simulink model "blocks"  (R2017b)
settings: Solver=VariableStepAuto  StartTime=0.0  StopTime=10.0  RelTol=1e-3
undefined symbols (not defined in the file or in its folder): environment
libraries: sharedtransform x1, aerolibnav x1
settings Model: Creator=Martin  LastModifiedBy=Martin

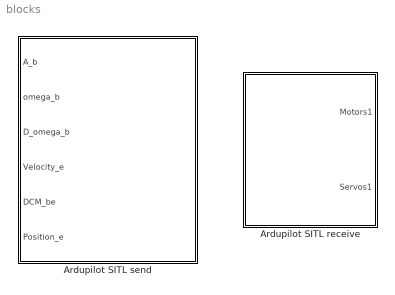
== system blocks ==
  Ardupilot SITL receive : Subsystem
  Ardupilot SITL send : Subsystem

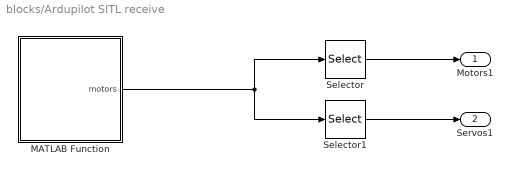
== system blocks/Ardupilot SITL receive ==
  MATLAB Function : MATLAB Function  TreatAsAtomicUnit=on  SystemSampleTime=0.02
  Selector : Selector  InputPortWidth=16  IndexOptions=Index vector (dialog)  Indices=sitl.output.motors  OutputSizes=1
  Selector1 : Selector  InputPortWidth=16  IndexOptions=Index vector (dialog)  Indices=sitl.output.servos  OutputSizes=1
  Motors1 : Outport
  Servos1 : Outport  Port=2
  wires:
  Selector1/1 -> Servos1/1
  Selector/1 -> Motors1/1
  MATLAB Function/1(motors) -> Selector1/1, Selector/1

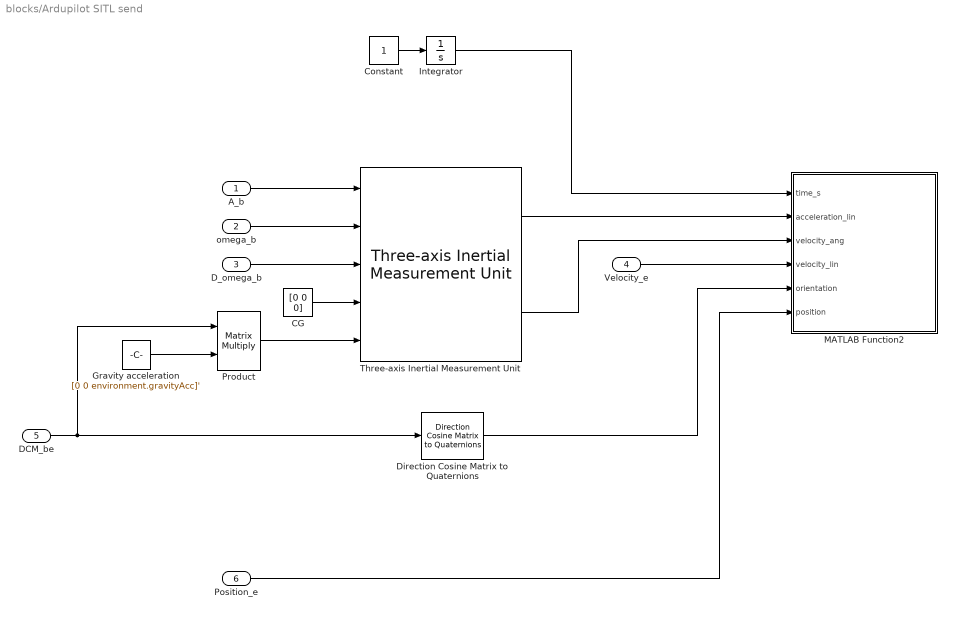
== system blocks/Ardupilot SITL send ==
  A_b : Inport
  omega_b : Inport  Port=2
  D_omega_b : Inport  Port=3
  Velocity_e : Inport  Port=4
  "DCM_be " : Inport  Port=5
  Position_e : Inport  Port=6
  CG : Constant  Value=[0 0 0]
  Constant : Constant
  Direction Cosine Matrix to Quaternions : sharedtransform/Direction Cosine Matrix  to Quaternions
      settings: SourceProductName=Aerospace Blockset  SourceProductBaseCode=AE
  Gravity acceleration : Constant  Value=[0 0 environment.gravityAcc]'
  Integrator : Integrator
  MATLAB Function2 : MATLAB Function  TreatAsAtomicUnit=on  SystemSampleTime=0.002
  Product : Product  Multiplication=Matrix(*)
  Three-axis Inertial Measurement Unit : aerolibnav/Three-axis Inertial Measurement Unit  units=Metric (MKS)  imu=[0 0 0]  i_Ts=0  dtype_a=off  w_a=190  z_a=0.707  a_sf_cc=[1 0 0; 0 1 0; 0 0 1]  a_bias=[0 0 0]  a_sat="[-inf  -inf  -inf  inf inf inf]"  dtype_g=off  w_g=190  z_g=0.707  g_sf_cc=[1 0 0; 0 1 0; 0 0 1]  g_bias=[0 0 0]  g_sens=[0 0 0]  g_sat="[-inf  -inf  -inf  inf inf inf]"  i_rand=off  i_seeds=[23093 23094 23095 23096 23097 23098]  i_pow=[0.001 0.001 0.001 0.0001 0.0001 0.0001]
  wires:
  omega_b/1 -> Three-axis Inertial Measurement Unit/2
  A_b/1 -> Three-axis Inertial Measurement Unit/1
  Constant/1 -> Integrator/1
  Integrator/1 -> MATLAB Function2/1(time_s)
  Position_e/1 -> MATLAB Function2/6(position)
  Velocity_e/1 -> MATLAB Function2/4(velocity_lin)
  CG/1 -> Three-axis Inertial Measurement Unit/4
  D_omega_b/1 -> Three-axis Inertial Measurement Unit/3
  Three-axis Inertial Measurement Unit/1 -> MATLAB Function2/2(acceleration_lin)
  Three-axis Inertial Measurement Unit/2 -> MATLAB Function2/3(velocity_ang)
  "DCM_be "/1 -> Direction Cosine Matrix to Quaternions/1, Product/1
  Direction Cosine Matrix to Quaternions/1 -> MATLAB Function2/5(orientation)
  Gravity acceleration/1 -> Product/2
  Product/1 -> Three-axis Inertial Measurement Unit/5

== matlab function blocks/Ardupilot SITL receive/MATLAB Function ==
  data: motors output
function motors = fcn()
motors = zeros(16 ,1);
coder.extrinsic('-sync:on','simReceive');
motors = simReceive();
end

== matlab function blocks/Ardupilot SITL send/MATLAB Function2 ==
  data: time_s input; acceleration_lin input; velocity_ang input; velocity_lin input; orientation input; position input
function fcn(time_s, acceleration_lin, velocity_ang, velocity_lin, orientation, position)
coder.extrinsic('-sync:on','simSend');
simSend(time_s, velocity_ang, velocity_lin, acceleration_lin, orientation, position);
